simulink model "Q1section2"  (R2019a)
settings: Solver=VariableStepAuto  StartTime=0.0  StopTime=100  RelTol=1e-3
settings Model: Creator=gal  LastModifiedBy=gal

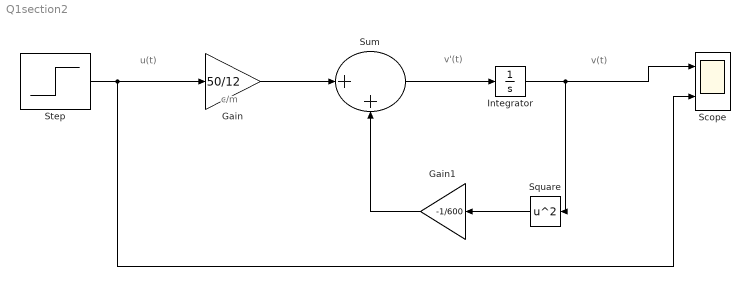
== system Q1section2 ==
  note: u(t)
  note: v'(t)
  note: v(t)
  note: c/m
  Gain : Gain  Gain=50/12
  Gain1 : Gain  Gain=-1/600
  Integrator : Integrator
  Scope : Scope  NumInputPorts=2
  Square : Math  Operator=square  SaturateOnIntegerOverflow=on
  Step : Step  Time=0  SampleTime=0
  Sum : Sum  Inputs=|++
  wires:
  Gain/1 -> Sum/1
  Sum/1 -> Integrator/1
  Gain1/1 -> Sum/2
  Square/1 -> Gain1/1
  Integrator/1 -> Square/1, Scope/1
  Step/1 -> Scope/2, Gain/1
